simulink model "Grid_VSI_Bo_test"  (Simulink 8.1)
settings: Solver=ode23t  StartTime=0.0  StopTime=20  MaxStep=1e-4  RelTol=1e-4  AbsTol=1e-5
InitFcn:
  | Vgllrms=120*sqrt(3);
  | 
  | Ivsi = 190;%190;%
  | 
  | L_grid=2e-3;%
  | R_grid= 0.2;%2;%
  | LLoad = 60e-3;
  | RLoad = 10;
  | CLoad = 250e-6;
  | 
  | kivsi = 3.2;%32;%
  | kpvsi= 1.5;%3;%
libraries: powerlib x38, simulink x1
settings Model: Creator=DongDong  LastModifiedBy=wenbo

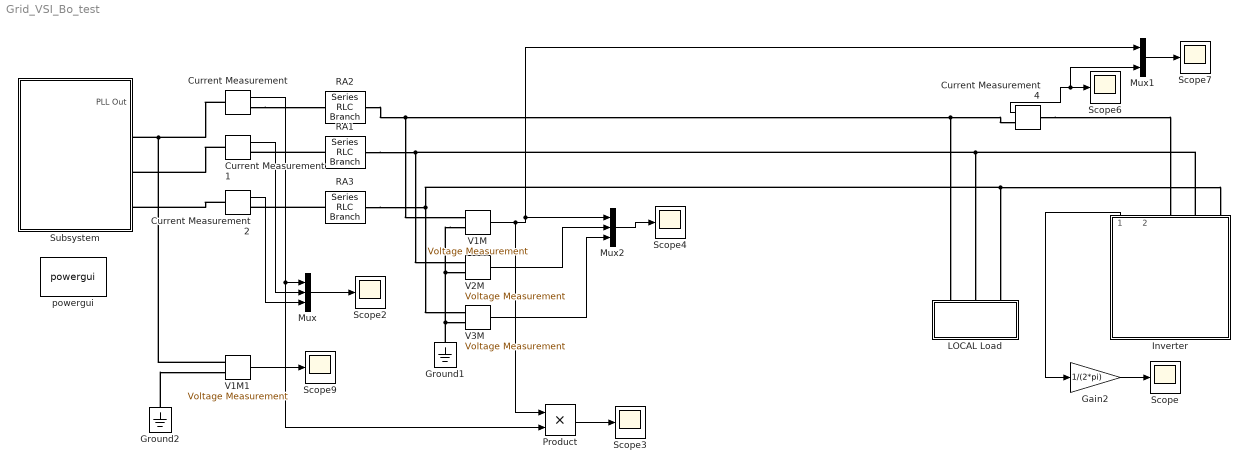
== system Grid_VSI_Bo_test ==
  Current Measurement{,1..2,4} (4 alike) : powerlib/Measurements/Current Measurement  PhasorSimulation=off  OutputType=Complex  PSBequivalent=0
  Gain2 : Gain  Gain=1/(2*pi)
  Ground1 : powerlib/Elements/Ground  LConnTagsString=a
  Ground2 : powerlib/Elements/Ground  LConnTagsString=a
  Inverter : Subsystem
  LOCAL Load : Subsystem
  Mux : Mux  Inputs=3
  Mux1 : Mux  Inputs=2
  Mux2 : Mux  Inputs=3
  Product : Product  RndMeth=Zero
  RA1 : powerlib/Elements/Series RLC Branch  LConnTagsString=__new0  RConnTagsString=__new0  BranchType=RL  Resistance=R_grid  Inductance=L_grid  SetiL0=off  InitialCurrent=0  Capacitance=1e-6  Setx0=off  InitialVoltage=0  Measurements=None
  RA2 : powerlib/Elements/Series RLC Branch  LConnTagsString=__new0  RConnTagsString=__new0  BranchType=RL  Resistance=R_grid  Inductance=L_grid  SetiL0=off  InitialCurrent=0  Capacitance=1e-6  Setx0=off  InitialVoltage=0  Measurements=None
  RA3 : powerlib/Elements/Series RLC Branch  LConnTagsString=__new0  RConnTagsString=__new0  BranchType=RL  Resistance=R_grid  Inductance=L_grid  SetiL0=off  InitialCurrent=0  Capacitance=1e-6  Setx0=off  InitialVoltage=0  Measurements=None
  Scope{,2..4,6..7,9} (7 alike) : Scope
      Scope settings: YMin=25  YMax=275  SaveName=f_vsi
      Scope2 settings: TimeRange=0.2371669915529565  YMin=-150  YMax=150  SaveName=IVSI
      Scope3 settings: TimeRange=0.2371669915529565  YMin=-42500  YMax=2500  SaveName=ScopeData3
      Scope4 settings: YMin=-1500  YMax=1500  SaveName=Vpcc
      Scope6 settings: TimeRange=0.2371669915529565  YMin=-100  YMax=100  SaveName=ScopeData6
      Scope7 settings: TimeRange=0.2371669915529565  YMin=-450  YMax=450  SaveName=ScopeData7
      Scope9 settings: TimeRange=0.2371669915529565  YMin=-225  YMax=225  SaveName=ScopeData9
  Subsystem : Subsystem
  V1M : powerlib/Measurements/Voltage Measurement  PhasorSimulation=off  OutputType=Complex  PSBequivalent=0
  V1M1 : powerlib/Measurements/Voltage Measurement  PhasorSimulation=off  OutputType=Complex  PSBequivalent=0
  V2M : powerlib/Measurements/Voltage Measurement  PhasorSimulation=off  OutputType=Complex  PSBequivalent=0
  V3M : powerlib/Measurements/Voltage Measurement  PhasorSimulation=off  OutputType=Complex  PSBequivalent=0
  powergui : powerlib/powergui  Priority=1  SimulationMode=Continuous  SolverType=Tustin  SampleTime=50e-6  frequency=60  SPID=off  DisableSnubberDevices=off  DisableRonSwitches=off  DisableVfSwitches=off  SwTol=0  Interpol=off  DisplayEquations=off  frequencyindice=0  Pbase=100e6  ErrMax=1e-4  Iterations=50  UnitsV=kV  UnitsW=MW  FunctionMessages=off  echomessages=off  HookPort=off  EnableUseOfTLC=off  x0status=blocks  RestoreLinks=warning  ResistiveCurrentMeasurement=off  Frange=[0:2:500]  Ylog=off  Xlog=on  ShowGrid=off  save=off  variable=ZData  ZoomFFT=on  StartTime=0.0  cycles=1  DisplayStyle=1  fundamental=60  FreqAxis=off  MaxFrequency=1000  frequencyindicesteady=1  RmsSteady=1  display=off  Ts=0  methode=off
  wires:
  Inverter/1(PLL Out) -> Gain2/1
  V1M/1 -> Product/1, Mux2/1, Mux1/1
  Current Measurement/1 -> Mux/1, Product/2
  Current Measurement1/1 -> Mux/2
  Current Measurement2/1 -> Mux/3
  Mux/1 -> Scope2/1
  Product/1 -> Scope3/1
  Current Measurement4/1 -> Scope6/1, Mux1/2
  Mux1/1 -> Scope7/1
  V1M1/1 -> Scope9/1
  Gain2/1 -> Scope/1
  Mux2/1 -> Scope4/1
  V2M/1 -> Mux2/2
  V3M/1 -> Mux2/3
  connections:
  RA2/LConn1 -- V1M/LConn1 -- Current Measurement4/RConn1 -- LOCAL Load/LConn1
  Inverter/RConn2 -- LOCAL Load/LConn2 -- RA1/LConn1 -- V2M/LConn1
  Inverter/RConn3 -- LOCAL Load/LConn3 -- RA3/LConn1 -- V3M/LConn1
  V1M/LConn2 -- Ground1/LConn1 -- V3M/LConn2 -- V2M/LConn2
  Current Measurement/RConn1 -- RA2/RConn1
  Current Measurement/LConn1 -- V1M1/LConn1 -- Subsystem/RConn1
  RA1/RConn1 -- Current Measurement1/RConn1
  Current Measurement1/LConn1 -- Subsystem/RConn2
  RA3/RConn1 -- Current Measurement2/RConn1
  Current Measurement2/LConn1 -- Subsystem/RConn3
  Current Measurement4/LConn1 -- Inverter/RConn1
  Ground2/LConn1 -- V1M1/LConn2

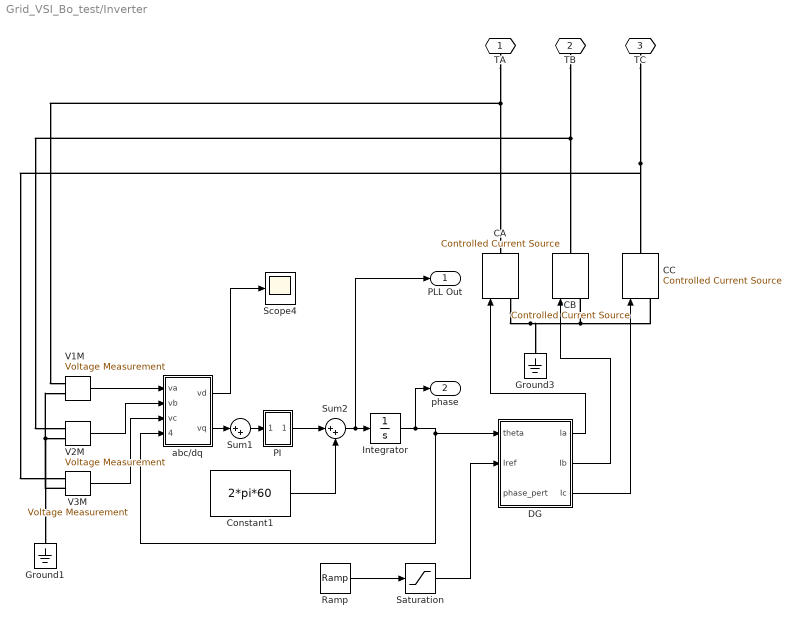
== system Grid_VSI_Bo_test/Inverter ==
  CA : powerlib/Electrical Sources/Controlled Current Source  Initialize=on  Source_Type=AC  Amplitude=0  Phase=0  Frequency=0  Measurements=None
  CB : powerlib/Electrical Sources/Controlled Current Source  Initialize=on  Source_Type=AC  Amplitude=0  Phase=0  Frequency=0  Measurements=None
  CC : powerlib/Electrical Sources/Controlled Current Source  Initialize=on  Source_Type=AC  Amplitude=0  Phase=0  Frequency=0  Measurements=None
  Constant1 : Constant  Value=2*pi*60
  DG : Subsystem
  Ground1 : powerlib/Elements/Ground  LConnTagsString=a
  Ground3 : powerlib/Elements/Ground  LConnTagsString=a
  Integrator : Integrator
  PI : Subsystem
  Ramp : simulink/Sources/Ramp  slope=50  start=2  X0=0
  Saturation : Saturate  UpperLimit=Ivsi  LowerLimit=-6
  Scope4 : Scope
      settings: TimeRange=0.2371669915529565  YMin=-200  YMax=200
  Sum1 : Sum  Inputs=|++
  Sum2 : Sum  Inputs=|++
  V1M : powerlib/Measurements/Voltage Measurement  PhasorSimulation=off  OutputType=Complex  PSBequivalent=0
  V2M : powerlib/Measurements/Voltage Measurement  PhasorSimulation=off  OutputType=Complex  PSBequivalent=0
  V3M : powerlib/Measurements/Voltage Measurement  PhasorSimulation=off  OutputType=Complex  PSBequivalent=0
  abc/dq : Subsystem
  TA : PMIOPort  Port=1  Side=Right
  TB : PMIOPort  Port=2  Side=Right
  TC : PMIOPort  Port=3  Side=Right
  PLL Out : Outport
  phase : Outport  Port=2
  wires:
  Integrator/1 -> phase/1, abc/dq/4(theta), DG/1(theta)
  Saturation/1 -> DG/2(Iref)
  Sum2/1 -> Integrator/1, PLL Out/1
  PI/1(out) -> Sum2/1
  Constant1/1 -> Sum2/2
  abc/dq/2(vq) -> Sum1/1
  Sum1/1 -> PI/1(in)
  DG/1(Ia) -> CA/1
  DG/2(Ib) -> CB/1
  DG/3(Ic) -> CC/1
  V1M/1 -> abc/dq/1(va)
  V2M/1 -> abc/dq/2(vb)
  V3M/1 -> abc/dq/3(vc)
  abc/dq/1(vd) -> Scope4/1
  Ramp/1 -> Saturation/1
  connections:
  CA/LConn1 -- CB/LConn1 -- CC/LConn1 -- Ground3/LConn1
  TA/RConn1 -- CA/RConn1 -- V1M/LConn1
  TB/RConn1 -- CB/RConn1 -- V2M/LConn1
  TC/RConn1 -- CC/RConn1 -- V3M/LConn1
  V3M/LConn2 -- Ground1/LConn1 -- V1M/LConn2 -- V2M/LConn2

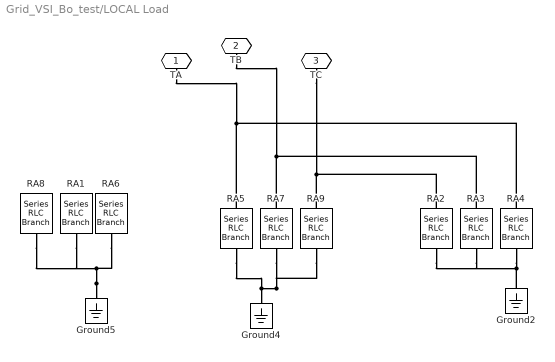
== system Grid_VSI_Bo_test/LOCAL Load ==
  Ground2 : powerlib/Elements/Ground  LConnTagsString=a
  Ground4 : powerlib/Elements/Ground  LConnTagsString=a
  Ground5 : powerlib/Elements/Ground  LConnTagsString=a
  RA1 : powerlib/Elements/Series RLC Branch  LConnTagsString=__new0  RConnTagsString=__new0  BranchType=L  Resistance=0.01e-3  Inductance=LLoad  SetiL0=off  InitialCurrent=0  Capacitance=10e-6  Setx0=off  InitialVoltage=0  Measurements=None
  RA2 : powerlib/Elements/Series RLC Branch  LConnTagsString=__new0  RConnTagsString=__new0  BranchType=R  Resistance=RLoad  Inductance=1e-3  SetiL0=off  InitialCurrent=0  Capacitance=1e-6  Setx0=off  InitialVoltage=0  Measurements=None
  RA3 : powerlib/Elements/Series RLC Branch  LConnTagsString=__new0  RConnTagsString=__new0  BranchType=R  Resistance=RLoad  Inductance=1e-3  SetiL0=off  InitialCurrent=0  Capacitance=1e-6  Setx0=off  InitialVoltage=0  Measurements=None
  RA4 : powerlib/Elements/Series RLC Branch  LConnTagsString=__new0  RConnTagsString=__new0  BranchType=R  Resistance=RLoad  Inductance=1e-3  SetiL0=off  InitialCurrent=0  Capacitance=1e-6  Setx0=off  InitialVoltage=0  Measurements=None
  RA5 : powerlib/Elements/Series RLC Branch  LConnTagsString=__new0  RConnTagsString=__new0  BranchType=C  Resistance=0.01e-3  Inductance=80e-3  SetiL0=off  InitialCurrent=0  Capacitance=CLoad  Setx0=off  InitialVoltage=0  Measurements=None
  RA6 : powerlib/Elements/Series RLC Branch  LConnTagsString=__new0  RConnTagsString=__new0  BranchType=L  Resistance=0.01e-3  Inductance=LLoad  SetiL0=off  InitialCurrent=0  Capacitance=10e-6  Setx0=off  InitialVoltage=0  Measurements=None
  RA7 : powerlib/Elements/Series RLC Branch  LConnTagsString=__new0  RConnTagsString=__new0  BranchType=C  Resistance=0.01e-3  Inductance=80e-3  SetiL0=off  InitialCurrent=0  Capacitance=CLoad  Setx0=off  InitialVoltage=0  Measurements=None
  RA8 : powerlib/Elements/Series RLC Branch  LConnTagsString=__new0  RConnTagsString=__new0  BranchType=L  Resistance=0.01e-3  Inductance=LLoad  SetiL0=off  InitialCurrent=0  Capacitance=10e-6  Setx0=off  InitialVoltage=0  Measurements=None
  RA9 : powerlib/Elements/Series RLC Branch  LConnTagsString=__new0  RConnTagsString=__new0  BranchType=C  Resistance=0.01e-3  Inductance=80e-3  SetiL0=off  InitialCurrent=0  Capacitance=CLoad  Setx0=off  InitialVoltage=0  Measurements=None
  TA : PMIOPort  Port=1  Side=Left
  TB : PMIOPort  Port=2  Side=Left
  TC : PMIOPort  Port=3  Side=Left
  connections:
  Ground2/LConn1 -- RA2/RConn1 -- RA3/RConn1 -- RA4/RConn1
  Ground4/LConn1 -- RA5/RConn1 -- RA9/RConn1 -- RA7/RConn1
  Ground5/LConn1 -- RA6/RConn1 -- RA1/RConn1 -- RA8/RConn1
  TA/RConn1 -- RA5/LConn1 -- RA4/LConn1
  TB/RConn1 -- RA7/LConn1 -- RA3/LConn1
  TC/RConn1 -- RA9/LConn1 -- RA2/LConn1

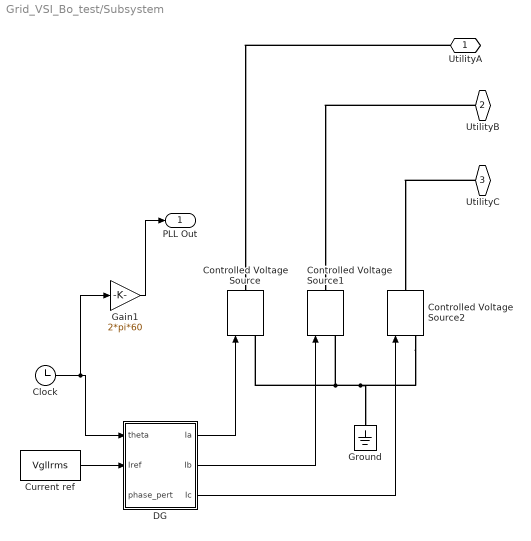
== system Grid_VSI_Bo_test/Subsystem ==
  Clock : Clock
  Controlled Voltage Source : powerlib/Electrical Sources/Controlled Voltage Source  Initialize=on  Source_Type=AC  Amplitude=0  Phase=0  Frequency=0  Measurements=None
  Controlled Voltage Source1 : powerlib/Electrical Sources/Controlled Voltage Source  Initialize=on  Source_Type=AC  Amplitude=0  Phase=0  Frequency=0  Measurements=None
  Controlled Voltage Source2 : powerlib/Electrical Sources/Controlled Voltage Source  Initialize=on  Source_Type=AC  Amplitude=0  Phase=0  Frequency=0  Measurements=None
  Current ref : Constant  Value=Vgllrms
  DG : Subsystem
  Gain1 : Gain  Gain=2*pi*60
  Ground : powerlib/Elements/Ground  LConnTagsString=a
  UtilityA : PMIOPort  Port=1  Side=Right
  UtilityB : PMIOPort  Port=2  Side=Right
  UtilityC : PMIOPort  Port=3  Side=Right
  PLL Out : Outport
  wires:
  DG/1(Ia) -> Controlled Voltage Source/1
  DG/2(Ib) -> Controlled Voltage Source1/1
  DG/3(Ic) -> Controlled Voltage Source2/1
  ? -> DG/3(phase_pert)
  Current ref/1 -> DG/2(Iref)
  Clock/1 -> DG/1(theta), Gain1/1
  Gain1/1 -> PLL Out/1
  connections:
  Controlled Voltage Source2/LConn1 -- Controlled Voltage Source/LConn1 -- Controlled Voltage Source1/LConn1 -- Ground/LConn1
  UtilityC/RConn1 -- Controlled Voltage Source2/RConn1
  UtilityB/RConn1 -- Controlled Voltage Source1/RConn1
  UtilityA/RConn1 -- Controlled Voltage Source/RConn1

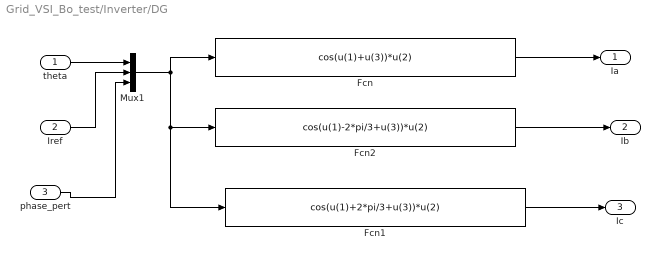
== system Grid_VSI_Bo_test/Inverter/DG ==
  theta : Inport
  Iref : Inport  Port=2
  phase_pert : Inport  Port=3
  Fcn : Fcn  Expr=cos(u(1)+u(3))*u(2)
  Fcn1 : Fcn  Expr=cos(u(1)+2*pi/3+u(3))*u(2)
  Fcn2 : Fcn  Expr=cos(u(1)-2*pi/3+u(3))*u(2)
  Mux1 : Mux  Inputs=3
  Ia : Outport
  Ib : Outport  Port=2
  Ic : Outport  Port=3
  wires:
  Fcn/1 -> Ia/1
  Fcn2/1 -> Ib/1
  Fcn1/1 -> Ic/1
  theta/1 -> Mux1/1
  Mux1/1 -> Fcn/1, Fcn2/1, Fcn1/1
  Iref/1 -> Mux1/2
  phase_pert/1 -> Mux1/3

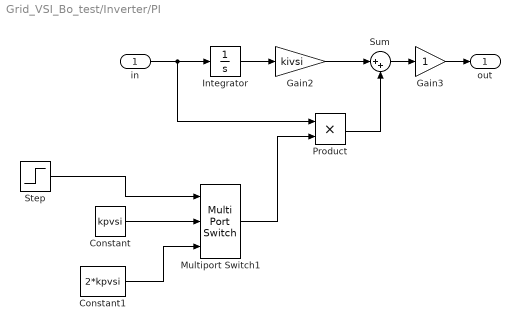
== system Grid_VSI_Bo_test/Inverter/PI ==
  in : Inport
  Constant : Constant  Value=kpvsi
  Constant1 : Constant  Value=2*kpvsi
  Gain2 : Gain  Gain=kivsi
  Gain3 : Gain
  Integrator : Integrator
  Multiport Switch1 : MultiPortSwitch  DataPortOrder=Zero-based contiguous  Inputs=2  DiagnosticForDefault=None
  Product : Product
  Step : Step  Time=10  SampleTime=0
  Sum : Sum  Inputs=|++
  out : Outport
  wires:
  in/1 -> Product/1, Integrator/1
  Integrator/1 -> Gain2/1
  Gain2/1 -> Sum/1
  Sum/1 -> Gain3/1
  Gain3/1 -> out/1
  Product/1 -> Sum/2
  Constant/1 -> Multiport Switch1/2
  Constant1/1 -> Multiport Switch1/3
  Multiport Switch1/1 -> Product/2
  Step/1 -> Multiport Switch1/1

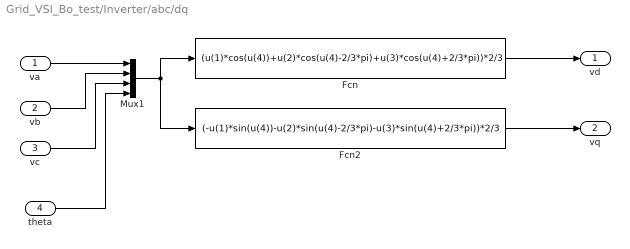
== system Grid_VSI_Bo_test/Inverter/abc/dq ==
  va : Inport
  vb : Inport  Port=2
  vc : Inport  Port=3
  theta : Inport  Port=4
  Fcn : Fcn  Expr=(u(1)*cos(u(4))+u(2)*cos(u(4)-2/3*pi)+u(3)*cos(u(4)+2/3*pi))*2/3
  Fcn2 : Fcn  Expr=(-u(1)*sin(u(4))-u(2)*sin(u(4)-2/3*pi)-u(3)*sin(u(4)+2/3*pi))*2/3
  Mux1 : Mux
  vd : Outport
  vq : Outport  Port=2
  wires:
  Mux1/1 -> Fcn/1, Fcn2/1
  va/1 -> Mux1/1
  vb/1 -> Mux1/2
  vc/1 -> Mux1/3
  theta/1 -> Mux1/4
  Fcn/1 -> vd/1
  Fcn2/1 -> vq/1

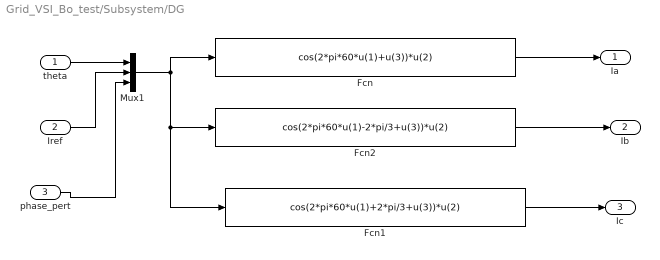
== system Grid_VSI_Bo_test/Subsystem/DG ==
  theta : Inport
  Iref : Inport  Port=2
  phase_pert : Inport  Port=3
  Fcn : Fcn  Expr=cos(2*pi*60*u(1)+u(3))*u(2)
  Fcn1 : Fcn  Expr=cos(2*pi*60*u(1)+2*pi/3+u(3))*u(2)
  Fcn2 : Fcn  Expr=cos(2*pi*60*u(1)-2*pi/3+u(3))*u(2)
  Mux1 : Mux  Inputs=3
  Ia : Outport
  Ib : Outport  Port=2
  Ic : Outport  Port=3
  wires:
  Fcn/1 -> Ia/1
  Fcn2/1 -> Ib/1
  Fcn1/1 -> Ic/1
  theta/1 -> Mux1/1
  Mux1/1 -> Fcn/1, Fcn2/1, Fcn1/1
  Iref/1 -> Mux1/2
  phase_pert/1 -> Mux1/3
